simulink model "demo1"  (R2022a)
settings: Solver=VariableStepAuto  StartTime=0.0  StopTime=400  FixedStep=0.01  RelTol=1e-3
undefined symbols (not defined in the file or in its folder): datCar
libraries: slpidlib x1
settings Model: Creator=swami  LastModifiedBy=yaggi
settings SolverCC: AlgebraicLoopSolver=TrustRegion
settings DebuggingCC: UnconnectedInputMsg=warning  UnconnectedOutputMsg=warning  UnconnectedLineMsg=warning  SFMachineParentedDataDiag=warning

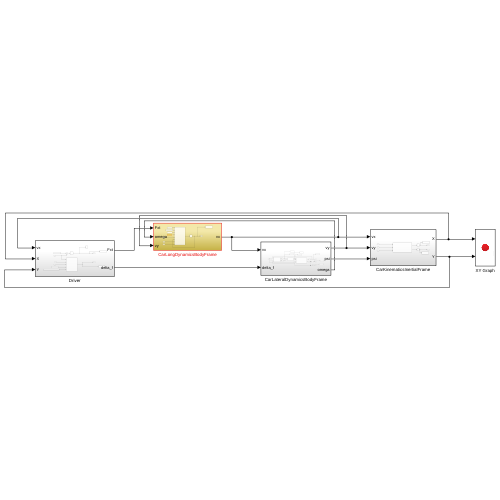
[thumbnail: Simulink's stored preview of the top-level diagram]
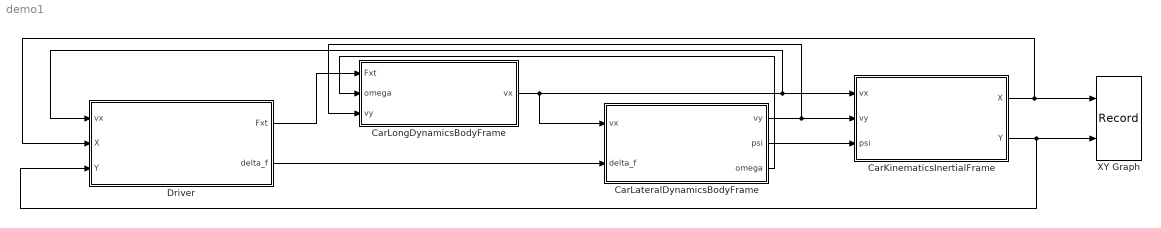
== system demo1 ==
  CarKinematicsInertialFrame : Subsystem
  CarLateralDynamicsBodyFrame : Subsystem
  CarLongDynamicsBodyFrame : Subsystem
  Driver : Subsystem
  XY Graph : Record  FileSettingsInternal="{\"entries\":[{\"content\":{\"excelSettings\":{\"content\":{},\"type\":\"Streamout.ExcelSettings\"}},\"type\":\"Streamout.FileSettingStorage\",\"uuid\":\"5896385b-20b2-444a-a4d6-ba6b82046aef\"}],\"packageUris\":[\"http://schema.mathworks.com/mf0/streamout_blocks/R2020a\"],\"version\":\"1.0\"}"  Layout=[1 1]  SignalsInternal="{\"entries\":[{\"content\":{\"signals\":[{\"content\":{\"blockPath\":[\"demo1/XY Graph\"],\"channel\":[],\"dimensions\":[1],\"domain\":\"demo1/XY Graph\",\"lineColor\":\"#a2142f\",\"plots\":[1],\"port\":1,\"sid\":[\"\"],\"signalID\":147,\"signalName\":\"CarKinematicsInertialFrame:1\"},\"type\":\"RecordBlkView.Signal\",\"uuid\":\"763fdaf7-82c6-41ca-8ae1-d419931e1d29\"},{\"content\":{\"blockPath\":[\"demo1/XY Graph\"],\"channel\":[],\"dimensions\":[1],\"domain\":\"demo1/XY Graph\",\"lineColor\":\"#139fff\",\"plots\":[1],\"port\":2,\"sid\":[\"\"],\"signalID\":151,\"signalName\":\"CarKinematicsInertialFrame:2\"},\"type\":\"RecordBlkView.Signal\",\"uuid\":\"faa157bf-e73a-47a4-8971-e997bf010f82\"}]},\"type\":\"RecordBlkView.InputSignals\",\"uuid\":\"92629f64-3519-4260-9b1f-879277dc4920\"}],\"packageUris\":[\"http://schema.mathworks.com/mf0/streamout_blocks/R2020a\"],\"version\":\"1.0\"}"  VisualizationBindings="{\"xyplotplugin\":{\"info\":[{\"series\":[{\"bindingParametersList\":[{\"parameter\":\"X-Axis\",\"signalID\":147,\"signalName\":\"CarKinematicsInertialFrame:1\"},{\"parameter\":\"Y-Axis\",\"signalID\":151,\"signalName\":\"CarKinematicsInertialFrame:2\"}],\"seriesID\":1469}],\"subplotID\":1}]}}"  CompatibilityTag=XY  st=-1
  wires:
  CarLongDynamicsBodyFrame/1(vx) -> CarLateralDynamicsBodyFrame/1(vx), Driver/1(vx), CarKinematicsInertialFrame/1(vx)
  CarLateralDynamicsBodyFrame/1(vy) -> CarLongDynamicsBodyFrame/3(vy), CarKinematicsInertialFrame/2(vy)
  CarLateralDynamicsBodyFrame/2(psi) -> CarKinematicsInertialFrame/3(psi)
  CarKinematicsInertialFrame/1(X) -> Driver/2("X "), XY Graph/1
  CarKinematicsInertialFrame/2(Y) -> Driver/3(Y), XY Graph/2
  Driver/2(delta_f) -> CarLateralDynamicsBodyFrame/2(delta_f)
  Driver/1(Fxt) -> CarLongDynamicsBodyFrame/1("Fxt ")
  CarLateralDynamicsBodyFrame/3(omega) -> CarLongDynamicsBodyFrame/2(omega)

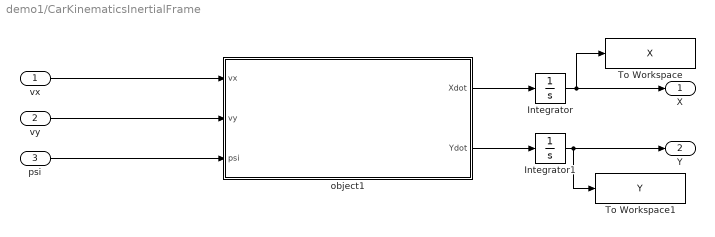
== system demo1/CarKinematicsInertialFrame ==
  vx : Inport
  vy : Inport  Port=2
  psi : Inport  Port=3
  Integrator : Integrator  InitialCondition=datCar.init.X0
  Integrator1 : Integrator  InitialCondition=datCar.init.Y0
  To Workspace : ToWorkspace  VariableName=X  SaveFormat=Timeseries  SampleTime=-1
  To Workspace1 : ToWorkspace  VariableName=Y  SaveFormat=Timeseries  SampleTime=-1
  object1 : MATLAB Function  TreatAsAtomicUnit=on  mask{obj=datCar}
      mask prompts: obj "obj structure"
  X : Outport
  Y : Outport  Port=2
  wires:
  object1/1(Xdot) -> Integrator/1
  object1/2(Ydot) -> Integrator1/1
  Integrator/1 -> To Workspace/1, X/1
  Integrator1/1 -> To Workspace1/1, Y/1
  vx/1 -> object1/1(vx)
  vy/1 -> object1/2(vy)
  psi/1 -> object1/3(psi)

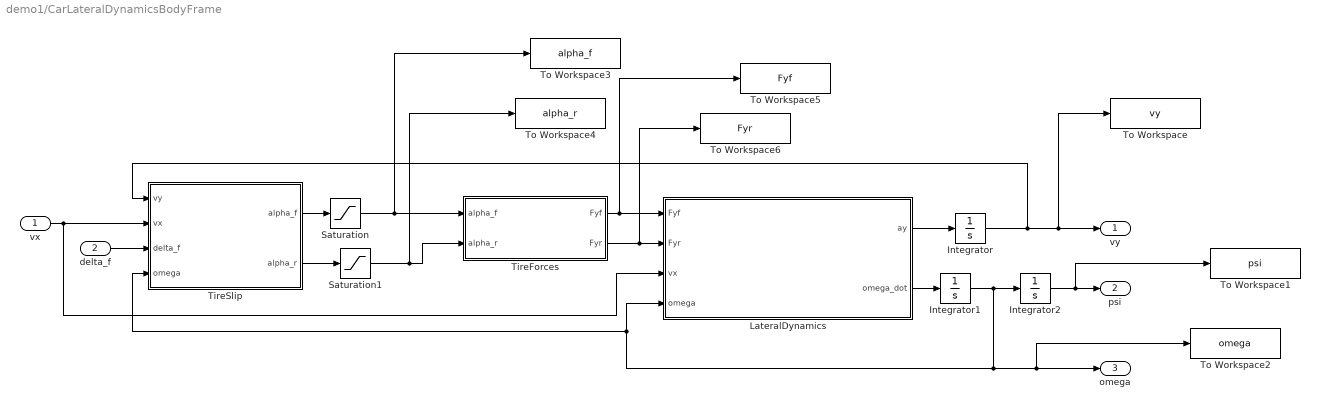
== system demo1/CarLateralDynamicsBodyFrame ==
  vx : Inport
  delta_f : Inport  Port=2
  Integrator : Integrator  InitialCondition=datCar.init.vy0
  Integrator1 : Integrator  InitialCondition=datCar.init.omega0
  Integrator2 : Integrator  InitialCondition=datCar.init.psi0
  LateralDynamics : MATLAB Function  TreatAsAtomicUnit=on  mask{obj=datCar}
      mask prompts: obj "obj structure"
  Saturation : Saturate  UpperLimit=datCar.maxAlpha  LowerLimit=-datCar.maxAlpha
  Saturation1 : Saturate  UpperLimit=datCar.maxAlpha  LowerLimit=-datCar.maxAlpha
  TireForces : MATLAB Function  TreatAsAtomicUnit=on  mask{obj=datCar}
      mask prompts: obj "obj structure"
  TireSlip : MATLAB Function  TreatAsAtomicUnit=on  mask{obj=datCar}
      mask prompts: obj "obj structure"
  To Workspace : ToWorkspace  VariableName=vy  SaveFormat=Timeseries  SampleTime=-1
  To Workspace1 : ToWorkspace  VariableName=psi  SaveFormat=Timeseries  SampleTime=-1
  To Workspace2 : ToWorkspace  VariableName=omega  SaveFormat=Timeseries  SampleTime=-1
  To Workspace3 : ToWorkspace  VariableName=alpha_f  SaveFormat=Timeseries  SampleTime=-1
  To Workspace4 : ToWorkspace  VariableName=alpha_r  SaveFormat=Timeseries  SampleTime=-1
  To Workspace5 : ToWorkspace  VariableName=Fyf  SaveFormat=Timeseries  SampleTime=-1
  To Workspace6 : ToWorkspace  VariableName=Fyr  SaveFormat=Timeseries  SampleTime=-1
  vy : Outport
  psi : Outport  Port=2
  omega : Outport  Port=3
  wires:
  LateralDynamics/1(ay) -> Integrator/1
  Integrator/1 -> TireSlip/1(vy), To Workspace/1, vy/1
  LateralDynamics/2(omega_dot) -> Integrator1/1
  Integrator1/1 -> TireSlip/4(omega), LateralDynamics/4(omega), To Workspace2/1, omega/1, Integrator2/1
  Integrator2/1 -> To Workspace1/1, psi/1
  TireSlip/1(alpha_f) -> Saturation/1
  TireSlip/2(alpha_r) -> Saturation1/1
  vx/1 -> LateralDynamics/3(vx), TireSlip/2(vx)
  delta_f/1 -> TireSlip/3(delta_f)
  TireForces/1(Fyf) -> To Workspace5/1, LateralDynamics/1(Fyf)
  TireForces/2(Fyr) -> To Workspace6/1, LateralDynamics/2(Fyr)
  Saturation/1 -> To Workspace3/1, TireForces/1(alpha_f)
  Saturation1/1 -> To Workspace4/1, TireForces/2(alpha_r)

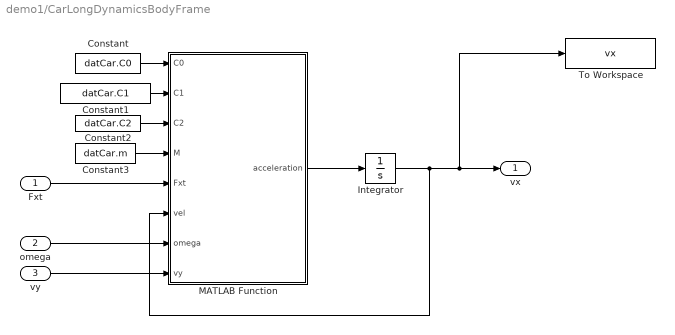
== system demo1/CarLongDynamicsBodyFrame ==
  "Fxt " : Inport
  omega : Inport  Port=2
  vy : Inport  Port=3
  Constant : Constant  Value=datCar.C0
  Constant1 : Constant  Value=datCar.C1
  Constant2 : Constant  Value=datCar.C2
  Constant3 : Constant  Value=datCar.m
  Integrator : Integrator  InitialCondition=datCar.init.vx0  LimitOutput=on  LowerSaturationLimit=0
  MATLAB Function : MATLAB Function  TreatAsAtomicUnit=on
  To Workspace : ToWorkspace  VariableName=vx  SaveFormat=Timeseries  SampleTime=-1
  vx : Outport  VectorParamsAs1DForOutWhenUnconnected=off
  wires:
  Constant1/1 -> MATLAB Function/2(C1)
  Constant/1 -> MATLAB Function/1(C0)
  MATLAB Function/1(acceleration) -> Integrator/1
  Constant2/1 -> MATLAB Function/3(C2)
  Constant3/1 -> MATLAB Function/4(M)
  "Fxt "/1 -> MATLAB Function/5(Fxt)
  Integrator/1 -> To Workspace/1, vx/1, MATLAB Function/6(vel)
  omega/1 -> MATLAB Function/7(omega)
  vy/1 -> MATLAB Function/8(vy)

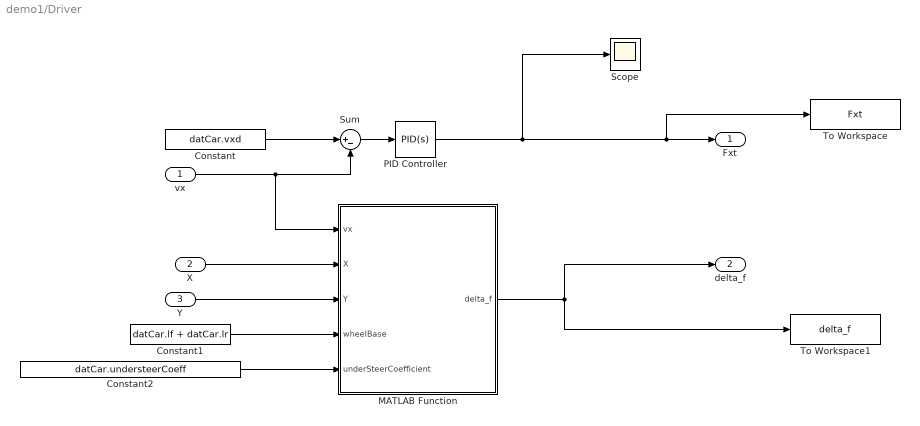
== system demo1/Driver ==
  vx : Inport
  "X " : Inport  Port=2
  Y : Inport  Port=3
  Constant : Constant  Value=datCar.vxd
  Constant1 : Constant  Value=datCar.lf + datCar.lr
  Constant2 : Constant  Value=datCar.understeerCoeff
  MATLAB Function : MATLAB Function  TreatAsAtomicUnit=on
  PID Controller : slpidlib/PID Controller  Controller=PID  Form=Parallel  TimeDomain=Continuous-time  UseExternalTs=off  SampleTime=-1  IntegratorMethod=Forward Euler  FilterMethod=Forward Euler  ControllerParametersSource=internal  P=1000  I=1  UseKiTs=off  D=0  N=100  UseFilter=on  TunerSelectOption=Transfer Function Based (PID Tuner App)  InitialConditionSource=internal  InitialConditionForIntegrator=0  InitialConditionForFilter=0  DifferentiatorICPrevScaledInput=0  ExternalReset=none  TrackingMode=off  Kt=1  LimitOutput=off  SatLimitsSource=internal  UpperSaturationLimit=inf  LowerSaturationLimit=-inf  LinearizeAsGain=on  AntiWindupMode=none  Kb=1  POutMin=[]  POutMax=[]  IOutMin=[]  IOutMax=[]  DOutMin=[]  DOutMax=[]  NOutMin=[]  NOutMax=[]  SumOutMin=[]  SumOutMax=[]  SaturationOutMin=[]  SaturationOutMax=[]  PParamMin=[]  PParamMax=[]  IParamMin=[]  IParamMax=[]  DParamMin=[]  DParamMax=[]  NParamMin=[]  NParamMax=[]  KbParamMin=[]  KbParamMax=[]  KtParamMin=[]  KtParamMax=[]  KbOutMin=[]  KbOutMax=[]  KtOutMin=[]  KtOutMax=[]  IntegratorOutMin=[]  IntegratorOutMax=[]  FilterOutMin=[]  FilterOutMax=[]  SumI1OutMin=[]  SumI1OutMax=[]  SumI2OutMin=[]  SumI2OutMax=[]  SumI3OutMin=[]  SumI3OutMax=[]  SumI4OutMin=[]  SumI4OutMax=[]  SumDOutMin=[]  SumDOutMax=[]  DifferentiatorOutMin=[]  DifferentiatorOutMax=[]  FilterDiffOutCoefMin=[]  FilterDiffOutCoefMax=[]  ReciprocalOutMin=[]  ReciprocalOutMax=[]  SumDenOutMin=[]  SumDenOutMax=[]  SumNumOutMin=[]  SumNumOutMax=[]  DivideOutMin=[]  DivideOutMax=[]  UdiffTsProdOutMin=[]  UdiffTsProdOutMax=[]  NTsProdOutMin=[]  NTsProdOutMax=[]  UintegralTsProdOutMin=[]  UintegralTsProdOutMax=[]  UngainTsProdOutMin=[]  UngainTsProdOutMax=[]  IntegratorContinuousStateAttributes=''  IntegratorStateMustResolveToSignalObject=off  IntegratorRTWStateStorageClass=Auto  FilterContinuousStateAttributes=''  FilterStateMustResolveToSignalObject=off  FilterRTWStateStorageClass=Auto  ParallelPVariant=InternalParameters  IdealPVariant=Disabled  IVariant=InternalParameters  DVariant=InternalParameters  IntegratorVariant=Continuous  SatVariant=Disabled  AWVariant=Passthrough  PCopyVariant=Disabled  TRVariant=Disabled  FdbkBlocksVariant=Forward  IdealPFdbkVariant=Disabled  SatFdbkVariant=Disabled  DerivativeFilterVariant=ContFilter  NVariant=InternalParameters  NCopyVariant=Disabled  FilterICVariant=InternalICsFilter  IntegratorICVariant=InternalICs  ExternalResetVariant=Disabled  TRSumVariant=Passthrough  SumFdbkVariant=Disabled  SumVariant=Sum_PID  TsampFilterVariant=InternalTs  TsampNgainVariant=Passthrough  TsampIntegralVariant=Passthrough  ExternalSaturationOutDataTypeStr=Inherit: Same as second input  aMode=0
  Scope : Scope
  Sum : Sum  Inputs=|+-
  To Workspace : ToWorkspace  VariableName=Fxt  SaveFormat=Timeseries  SampleTime=-1
  To Workspace1 : ToWorkspace  VariableName=delta_f  SaveFormat=Timeseries  SampleTime=-1
  Fxt : Outport
  delta_f : Outport  Port=2  VectorParamsAs1DForOutWhenUnconnected=off
  wires:
  Constant/1 -> Sum/1
  vx/1 -> MATLAB Function/1(vx), Sum/2
  Sum/1 -> PID Controller/1
  PID Controller/1 -> Scope/1, To Workspace/1, Fxt/1
  "X "/1 -> MATLAB Function/2(X)
  Y/1 -> MATLAB Function/3(Y)
  MATLAB Function/1(delta_f) -> delta_f/1, To Workspace1/1
  Constant1/1 -> MATLAB Function/4(wheelBase)
  Constant2/1 -> MATLAB Function/5(underSteerCoefficient)

== matlab function demo1/CarKinematicsInertialFrame/object1 ==
  data: vx input; vy input; psi input size=1; Xdot output; Ydot output
function [Xdot, Ydot] = fcn(vx, vy, psi)
temp = TF(psi) * [vx;vy]; 
Xdot = temp(1);
Ydot = temp(2);
  
end

function y = TF(psi)
y = [cos(psi), sin(psi); -sin(psi), cos(psi)];
end

== matlab function demo1/CarLateralDynamicsBodyFrame/LateralDynamics ==
  data: Fyf input; Fyr input size=1; vx input; omega input; ay output; obj parameter; omega_dot output
function [ay, omega_dot] = fcn(Fyf, Fyr, vx, omega, obj)

Fy = Fyf + Fyr;
ay = Fy / obj.m - omega * vx;
        
M  = Fyf * obj.lf - Fyr * obj.lr;        
omega_dot = M / obj.I;        

end

== matlab function demo1/CarLongDynamicsBodyFrame/MATLAB Function ==
  data: C0 input; acceleration output; C1 input; C2 input; M input; Fxt input; vel input; omega input; vy input
function acceleration   = vehicle(C0,C1,C2,M,Fxt, vel, omega, vy)

acceleration = (Fxt-(C0+ C1*vel + C2*(vel)^2))/M + omega * vy;

== matlab function demo1/Driver/MATLAB Function ==
  data: vx input; X input; delta_f output; Y input; wheelBase input; underSteerCoefficient input
function delta_f   = latControl(vx,X,Y,wheelBase, underSteerCoefficient)

track_radius = 200;
track_length = 900;

track_seg1_x0 = 0;
track_seg1_y0 = 0;
track_seg1_x1 = track_length;
track_seg1_y1 = 0;
track_seg2_x0 = track_seg1_x1;
track_seg2_y0 = track_seg1_y1;
track_seg2_x1 = track_seg2_x0;
track_seg2_y1 = track_seg2_y0 + 2 * track_radius;
track_seg3_x0 = track_seg2_x1;
track_seg3_y0 = track_seg2_y1;
track_seg3_x1 = track_seg3_x0 - track_length;
track_seg3_y1 = track_seg3_y0;
track_seg4_x0 = track_seg3_x1;
track_seg4_y0 = track_seg3_y1;
track_seg4_x1 = track_seg1_x0;
track_seg4_y1 = track_seg1_y0;

if X > track_seg1_x0
    if X > track_seg1_x1
        segment = 2;
    else
        if Y > (track_seg2_y0 + track_seg2_y1)/2
            segment = 3;
        else
            segment = 1;
        end
    end
else
    segment = 4;
end



switch(segment)
    case 1,
        delta_f = 0;
    case 2,
        delta_f = - (wheelBase / track_radius + 1 * underSteerCoefficient * vx^2);
    case 3,
        delta_f = 0;
    case 4
        delta_f = - (wheelBase / track_radius + 1 * underSteerCoefficient * vx^2);
    otherwise
        delta_f = 0;
end

== matlab function demo1/CarLateralDynamicsBodyFrame/TireSlip ==
  data: vy input size=1; vx input; delta_f input size=1; omega input; alpha_f output; obj parameter; alpha_r output
function [alpha_f, alpha_r] = fcn(vy,  vx, delta_f, omega, obj)


if abs(vx)> obj.vx_threshold1
      alpha_f = delta_f - (vy + omega * obj.lf) / vx;
      alpha_r = - (vy - omega * obj.lr) / vx;
else
      alpha_f = 0;
      alpha_r = 0;
end



end

== matlab function demo1/CarLateralDynamicsBodyFrame/TireForces ==
  data: alpha_f input; alpha_r input; Fyf output; obj parameter; Fyr output
function [Fyf, Fyr] = fcn(alpha_f, alpha_r, obj)

Fyf = min(obj.Fyfmax,obj.Calpha_f * alpha_f);
Fyr = min(obj.Fyrmax, obj.Calpha_r * alpha_r);
end
